simulink model "n4AP"  (Simulink 7.6)
settings: Solver=ode45  StartTime=0.0  StopTime=100  FixedStep=0.1  RelTol=1e-3
libraries: fuzblock x6
settings Model: Creator=federico  LastModifiedBy=federico

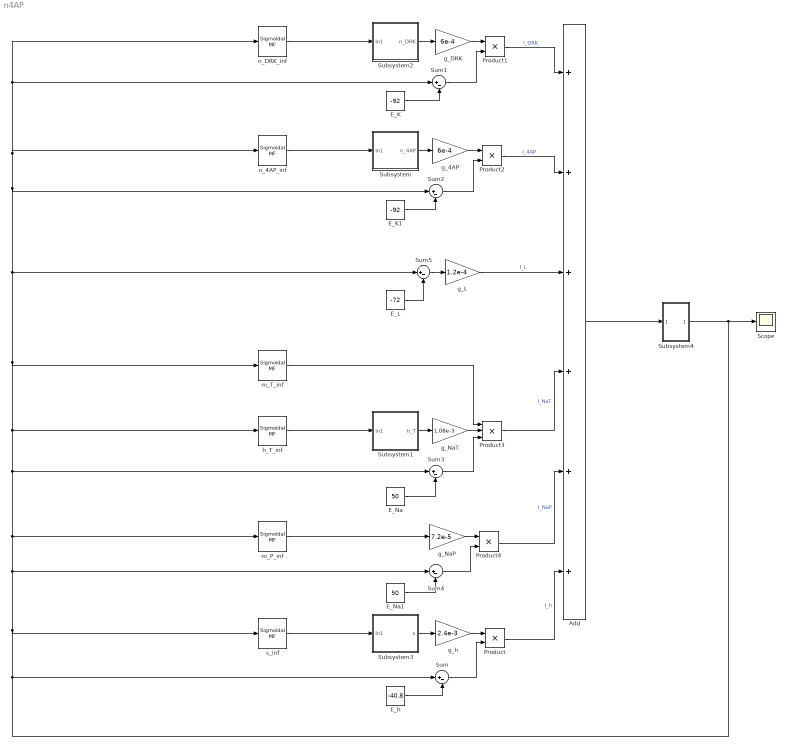
== system n4AP ==
  Add : Sum  Inputs=++++++
  E_K : Constant  Value=-92
  E_K1 : Constant  Value=-92
  E_L : Constant  Value=-72
  E_Na : Constant  Value=50
  E_Na1 : Constant  Value=50
  E_h : Constant  Value=-40.8
  Product{,1..2,4} (4 alike) : Product  RndMeth=Zero
  Product3 : Product  Inputs=3  RndMeth=Zero
  Scope : Scope
      settings: TimeRange=1.625  YMin=-20  YMax=140
  Subsystem : Subsystem
  Subsystem1 : Subsystem
  Subsystem2 : Subsystem
  Subsystem3 : Subsystem
  Subsystem4 : Subsystem
  Sum{,1..5} (6 alike) : Sum  Inputs=|+-
  g_4AP : Gain  Gain=6e-4
  g_DRK : Gain  Gain=6e-4
  g_L : Gain  Gain=1.2e-4
  g_NaP : Gain  Gain=7.2e-5
  g_NaT : Gain  Gain=1.08e-3
  g_h : Gain  Gain=2.4e-3
  h_T_inf : fuzblock/Membership  Functions/Sigmoidal MF  SystemSampleTime=-1  a=-1/7.1  c=-55
  m_P_inf : fuzblock/Membership  Functions/Sigmoidal MF  SystemSampleTime=-1  a=1/6.4  c=-50
  m_T_inf : fuzblock/Membership  Functions/Sigmoidal MF  SystemSampleTime=-1  a=1/4.3  c=-31.3
  n_4AP_inf : fuzblock/Membership  Functions/Sigmoidal MF  SystemSampleTime=-1  a=1/3.9  c=-43
  n_DRK_inf : fuzblock/Membership  Functions/Sigmoidal MF  SystemSampleTime=-1  a=1/12.9  c=-4.2
  s_inf : fuzblock/Membership  Functions/Sigmoidal MF  SystemSampleTime=-1  a=1/7.3  c=-105
  wires:
  n_4AP_inf/1 -> Subsystem/1(In1)
  n_DRK_inf/1 -> Subsystem2/1(In1)
  Product/1 -> Add/6  "I_h"
  g_DRK/1 -> Product1/1
  Sum1/1 -> Product1/2
  Product1/1 -> Add/1  "I_DRK"
  E_K/1 -> Sum1/2
  Subsystem2/1(n_DRK) -> g_DRK/1
  g_4AP/1 -> Product2/1
  Sum2/1 -> Product2/2
  Product2/1 -> Add/2  "I_4AP"
  E_K1/1 -> Sum2/2
  Subsystem/1(n_4AP) -> g_4AP/1
  Product3/1 -> Add/4  "I_NaT"
  g_NaP/1 -> Product4/1
  Sum4/1 -> Product4/2
  Product4/1 -> Add/5  "I_NaP"
  m_P_inf/1 -> g_NaP/1
  g_L/1 -> Add/3  "I_L"
  Sum5/1 -> g_L/1
  E_L/1 -> Sum5/2
  E_Na1/1 -> Sum4/2
  Add/1 -> Subsystem4/1(In1)
  Subsystem4/1(Out1) -> Sum5/1, n_4AP_inf/1, n_DRK_inf/1, Sum1/1, Sum2/1, m_T_inf/1, h_T_inf/1, Sum3/1, m_P_inf/1, Sum4/1, s_inf/1, Sum/1, Scope/1
  E_h/1 -> Sum/2
  Sum/1 -> Product/2
  g_h/1 -> Product/1
  Subsystem3/1(s) -> g_h/1
  s_inf/1 -> Subsystem3/1(In1)
  Sum3/1 -> Product3/3
  m_T_inf/1 -> Product3/1
  Subsystem1/1(h_T) -> g_NaT/1
  E_Na/1 -> Sum3/2
  g_NaT/1 -> Product3/2
  h_T_inf/1 -> Subsystem1/1(In1)

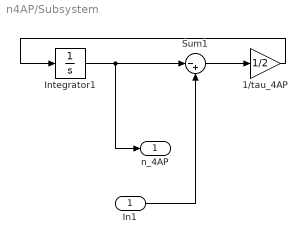
== system n4AP/Subsystem ==
  In1 : Inport
  1/tau_4AP : Gain  Gain=1/2
  Integrator1 : Integrator
  Sum1 : Sum  Inputs=|-+
  n_4AP : Outport
  wires:
  Integrator1/1 -> Sum1/1, n_4AP/1
  Sum1/1 -> 1/tau_4AP/1
  1/tau_4AP/1 -> Integrator1/1
  In1/1 -> Sum1/2

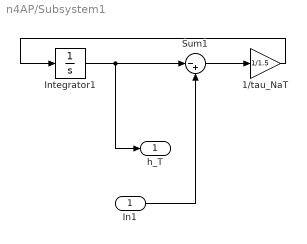
== system n4AP/Subsystem1 ==
  In1 : Inport
  1/tau_NaT : Gain  Gain=1/1.5
  Integrator1 : Integrator
  Sum1 : Sum  Inputs=|-+
  h_T : Outport
  wires:
  Integrator1/1 -> Sum1/1, h_T/1
  Sum1/1 -> 1/tau_NaT/1
  1/tau_NaT/1 -> Integrator1/1
  In1/1 -> Sum1/2

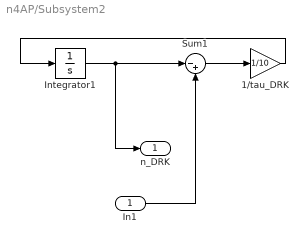
== system n4AP/Subsystem2 ==
  In1 : Inport
  1/tau_DRK : Gain  Gain=1/10
  Integrator1 : Integrator
  Sum1 : Sum  Inputs=|-+
  n_DRK : Outport
  wires:
  Integrator1/1 -> Sum1/1, n_DRK/1
  Sum1/1 -> 1/tau_DRK/1
  1/tau_DRK/1 -> Integrator1/1
  In1/1 -> Sum1/2

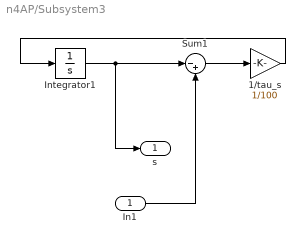
== system n4AP/Subsystem3 ==
  In1 : Inport
  1/tau_s : Gain  Gain=1/100
  Integrator1 : Integrator
  Sum1 : Sum  Inputs=|-+
  s : Outport
  wires:
  Integrator1/1 -> Sum1/1, s/1
  Sum1/1 -> 1/tau_s/1
  1/tau_s/1 -> Integrator1/1
  In1/1 -> Sum1/2

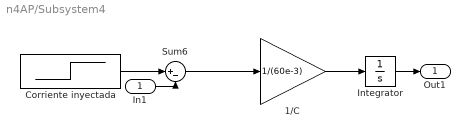
== system n4AP/Subsystem4 ==
  In1 : Inport
  1/C : Gain  Gain=1/(60e-3)
  Corriente inyectada : Step  SampleTime=0
  Integrator : Integrator
  Sum6 : Sum  Inputs=|+-
  Out1 : Outport
  wires:
  Sum6/1 -> 1/C/1
  1/C/1 -> Integrator/1
  Corriente inyectada/1 -> Sum6/1
  Integrator/1 -> Out1/1
  In1/1 -> Sum6/2
